simulink model "Dynamics"  (R2023a)
settings: Solver=FixedStepAuto  StartTime=0.0  StopTime=inf  FixedStep=0.001  EnableMultiTasking=on
libraries: sharedutil x32, sharedtransform x18, dspmtrx3 x12, matrix_library x6, simulink_extras x1, simulink x1
(part 1 of 6)
settings Model: VariantFading=off  Creator=Amir  LastModifiedBy=NGAI-LAPTOP
settings SolverCC: ZeroCrossAlgorithm=Adaptive  AutoInsertRateTranBlk=on
settings DataIOCC: LimitDataPoints=on  SaveFormat=Array  ReturnWorkspaceOutputs=off
settings OptimizationCC: LifeSpan=inf
settings DebuggingCC: UnconnectedInputMsg=warning  UnconnectedOutputMsg=warning  UnconnectedLineMsg=warning  SFUnexpectedBacktrackingDiag=warning  SFNoUnconditionalDefaultTransitionDiag=warning  SFExecutionAtInitializationDiag=none  ArithmeticOperatorsInVariantConditions=warning
settings HardwareCC: ProdBitPerPointer=32  ProdBitPerSizeT=32  ProdBitPerPtrDiffT=32  ProdLargestAtomicFloat=None  ProdIntDivRoundTo=Undefined  ProdEndianess=Unspecified  ProdWordSize=32  ProdHWDeviceType=32-bit Generic
settings ModelReferenceCC: PropagateSignalLabelsOutOfModel=off
settings SFSimCC: SimUseLocalCustomCode=off  CustomCodeUndefinedFunction=UseInterfaceOnly
settings RTWCC: RTWUseLocalCustomCode=off
settings CodeAppCC: StateflowObjectComments=on
settings GRTTargetCC: TargetLangStandard=C89/C90 (ANSI)
settings ConfigComp: CovMetricSettings=dw  CovSaveCumulativeToWorkspaceVar=on  CovSaveSingleToWorkspaceVar=on  CovExternalEMLEnable=off

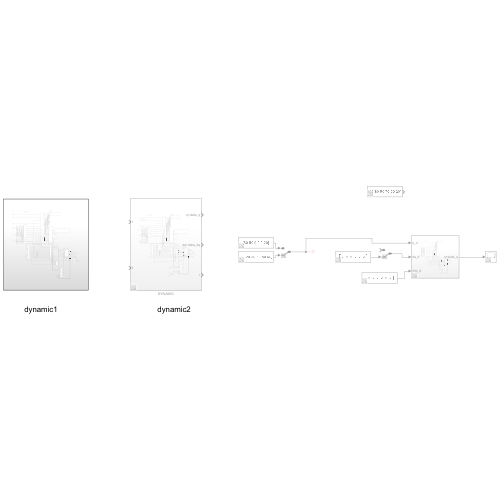
[thumbnail: Simulink's stored preview of the top-level diagram]
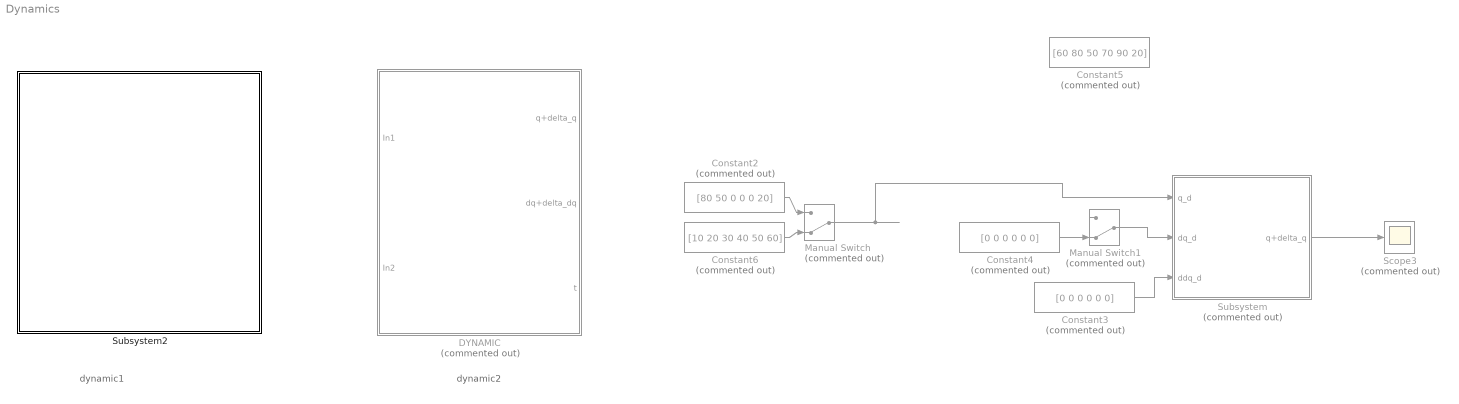
== system Dynamics ==
  note: dynamic1
  note: dynamic2
  Constant2 : Constant  Commented=on  Value=[80 50 0 0 0 20]
  Constant3 : Constant  Commented=on  Value=[0 0 0 0 0 0]
  Constant4 : Constant  Commented=on  Value=[0 0 0 0 0 0]
  Constant5 : Constant  Commented=on  Value=[60 80 50 70 90 20]
  Constant6 : Constant  Commented=on  Value=[10 20 30 40 50 60]
  DYNAMIC : Subsystem  Commented=on
  Manual Switch : ManualSwitch  Commented=on  CurrentSetting=0
  Manual Switch1 : ManualSwitch  Commented=on  CurrentSetting=0
  Scope3 : Scope  Commented=on
  Subsystem : Subsystem  Commented=on
  Subsystem2 : Subsystem
  wires:
  Subsystem/1(q+delta_q) -> Scope3/1
  Constant3/1 -> Subsystem/3(ddq_d)
  Constant2/1 -> Manual Switch/1
  Constant6/1 -> Manual Switch/2
  Manual Switch/1 -> Subsystem/1(q_d)
  Manual Switch1/1 -> Subsystem/2(dq_d)
  Constant4/1 -> Manual Switch1/2

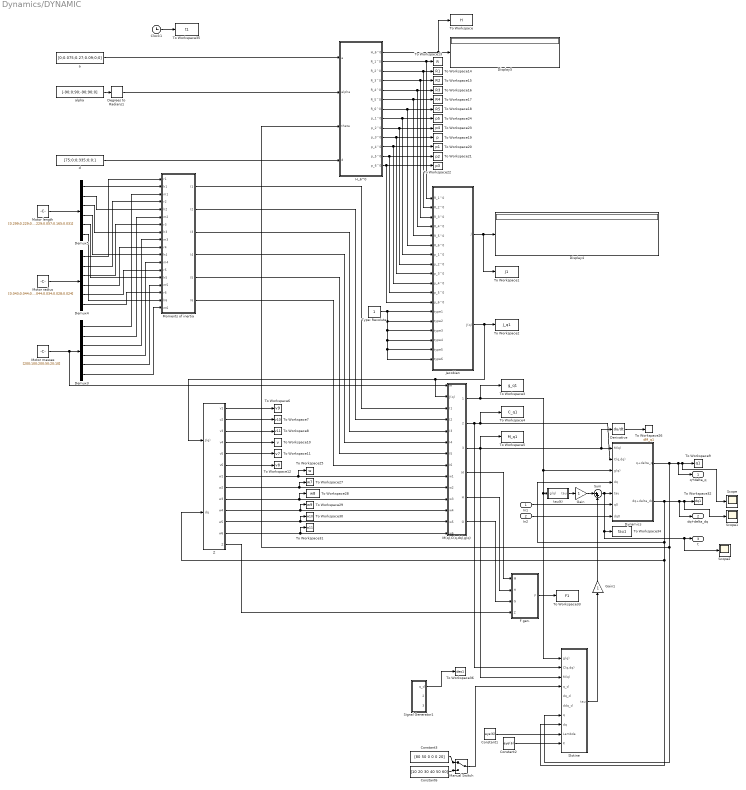
== system Dynamics/DYNAMIC ==
  In1 : Inport
  In2 : Inport  Port=2
  Clock1 : Clock
  Constant1 : Constant  Value=eye(6)
  Constant2 : Constant  Value=eye(6)
  Constant3 : Constant  Value=[80 50 0 0 0 20]
  Constant6 : Constant  Value=[10 20 30 40 50 60]
  Degrees to Radians1 : simulink_extras/Transformations/Degrees to Radians
  Demux3 : Demux  Outputs=6
  Demux4 : Demux  Outputs=6
  Demux5 : Demux  Outputs=6
  Derivative : Derivative
  Display4 : Display
  Display5 : Display
  Dynamics : Subsystem
  F gen. : Subsystem
  Gain : Gain
  Gain1 : Gain
  H_6^0 : Subsystem
  Jacobian : Subsystem
  M(q),C(q,dq),g(q) : Subsystem
  Manual Switch : ManualSwitch
  Moments of inertia : Subsystem
  Motor length : Constant  Value=[0.299;0.229;0.229;0.057;0.165;0.031]
  Motor masses : Constant  Value=[200;100;200;50;20;10]
  Motor radius : Constant  Value=[0.043;0.044;0.044;0.034;0.028;0.024]
  Scope : Scope
  Scope1 : Scope
  Scope2 : Scope
  Signal Generator1 : Subsystem
  Slotine : Subsystem
  Sum : Sum  Inputs=|++
  To Workspace : ToWorkspace  VariableName=H  SampleTime=-1
  To Workspace1 : ToWorkspace  VariableName=J1  SampleTime=-1
  To Workspace10 : ToWorkspace  VariableName=v  SampleTime=-1
  To Workspace11 : ToWorkspace  VariableName=v7  SampleTime=-1
  To Workspace12 : ToWorkspace  VariableName=v8  SampleTime=-1
  To Workspace13 : ToWorkspace  VariableName=R  SampleTime=-1
  To Workspace14 : ToWorkspace  VariableName=R1  SampleTime=-1
  To Workspace15 : ToWorkspace  VariableName=R2  SampleTime=-1
  To Workspace16 : ToWorkspace  VariableName=R3  SampleTime=-1
  To Workspace17 : ToWorkspace  VariableName=R4  SampleTime=-1
  To Workspace18 : ToWorkspace  VariableName=R5  SampleTime=-1
  To Workspace19 : ToWorkspace  VariableName=p  SampleTime=-1
  To Workspace2 : ToWorkspace  VariableName=J_q1  SampleTime=-1
  To Workspace20 : ToWorkspace  VariableName=p1  SampleTime=-1
  To Workspace21 : ToWorkspace  VariableName=p2  SampleTime=-1
  To Workspace22 : ToWorkspace  VariableName=p3  SampleTime=-1
  To Workspace23 : ToWorkspace  VariableName=p4  SampleTime=-1
  To Workspace24 : ToWorkspace  VariableName=p5  SampleTime=-1
  To Workspace25 : ToWorkspace  VariableName=w  SampleTime=-1
  To Workspace26 : ToWorkspace  VariableName=dM_q1  SampleTime=-1
  To Workspace27 : ToWorkspace  VariableName=w7  SampleTime=-1
  To Workspace28 : ToWorkspace  VariableName=w8  SampleTime=-1
  To Workspace29 : ToWorkspace  VariableName=w9  SampleTime=-1
  To Workspace3 : ToWorkspace  VariableName=g_q1  SampleTime=-1
  To Workspace30 : ToWorkspace  VariableName=w10  SampleTime=-1
  To Workspace31 : ToWorkspace  VariableName=w11  SampleTime=-1
  To Workspace32 : ToWorkspace  VariableName=dq1  SampleTime=-1
  To Workspace33 : ToWorkspace  VariableName=F1  SampleTime=-1
  To Workspace34 : ToWorkspace  VariableName=tau1  SampleTime=-1
  To Workspace35 : ToWorkspace  VariableName=t1  SampleTime=-1
  To Workspace36 : ToWorkspace  VariableName=des1  SampleTime=-1
  To Workspace4 : ToWorkspace  VariableName=C_q1  SampleTime=-1
  To Workspace5 : ToWorkspace  VariableName=M_q1  SampleTime=-1
  To Workspace6 : ToWorkspace  VariableName=v9  SampleTime=-1
  To Workspace7 : ToWorkspace  VariableName=v10  SampleTime=-1
  To Workspace8 : ToWorkspace  VariableName=v11  SampleTime=-1
  To Workspace9 : ToWorkspace  VariableName=q1  SampleTime=-1
  Type: Revolute : Constant
  Z : Subsystem
  a : Constant  Value=[0;0.075;0.27;0.09;0;0]
  alpha : Constant  Value=[-90;0;90;-90;90;0]
  d : Constant  Value=[75;0;0;335;0;0;]
  tau(t) : Subsystem
  q+delta_q : Outport
  dq+delta_dq : Outport  Port=2
  t : Outport  Port=3
  wires:
  Demux5/1 -> Moments of inertia/2(h1)
  Z/12(w6) -> To Workspace31/1, M(q),C(q,dq),g(q)/14(w6)
  Moments of inertia/6(I6) -> M(q),C(q,dq),g(q)/8(I6)
  Dynamics/2(dq+delta_dq) -> dq+delta_dq/1, Scope1/1, To Workspace32/1, Z/2(dq), Slotine/8(dq), Dynamics/4(dq)
  Z/11(w5) -> To Workspace30/1, M(q),C(q,dq),g(q)/13(w5)
  Moments of inertia/5(I5) -> M(q),C(q,dq),g(q)/7(I5)
  M(q),C(q,dq),g(q)/1(g(q)) -> Dynamics/3(g(q)), tau(t)/1(g(q)), Slotine/1(g(q)), To Workspace3/1
  Demux3/2 -> Moments of inertia/6(m2)
  Dynamics/1(q+delta_q) -> q+delta_q/1, Scope/1, To Workspace9/1, Slotine/7(q), H_6^0/3(theta)
  Moments of inertia/1(I1) -> M(q),C(q,dq),g(q)/3(I1)
  H_6^0/2(R_1^0) -> To Workspace13/1, Jacobian/1(R_1^0)
  In1/1 -> Dynamics/6(q0)
  Z/7(w1) -> To Workspace25/1, M(q),C(q,dq),g(q)/9(w1)
  Z/9(w3) -> To Workspace28/1, M(q),C(q,dq),g(q)/11(w3)
  Demux5/4 -> Moments of inertia/11(h4)
  Moments of inertia/4(I4) -> M(q),C(q,dq),g(q)/6(I4)
  Z/4(v4) -> To Workspace10/1
  H_6^0/12(p_5^0) -> To Workspace21/1, Jacobian/11(p_5^0)
  M(q),C(q,dq),g(q)/2(C(q,dq)) -> Slotine/2(C(q,dq)), To Workspace4/1, Dynamics/2(C(q,dq))
  Demux3/6 -> Moments of inertia/18(m6)
  Jacobian/2(J(q)) -> M(q),C(q,dq),g(q)/2(J(q)), Z/1(J(q)), To Workspace2/1
  H_6^0/11(p_4^0) -> To Workspace20/1, Jacobian/10(p_4^0)
  Demux3/3 -> Moments of inertia/9(m3)
  H_6^0/4(R_3^0) -> To Workspace15/1, Jacobian/3(R_3^0)
  Clock1/1 -> To Workspace35/1
  d/1 -> H_6^0/4(d)
  H_6^0/5(R_4^0) -> To Workspace16/1, Jacobian/4(R_4^0)
  Slotine/1(tau) -> Gain1/1
  Demux4/6 -> Moments of inertia/16(r6)
  H_6^0/1(H_6^0) -> To Workspace/1, Display5/1
  In2/1 -> Dynamics/7(dq0)
  H_6^0/8(p_1^0) -> Jacobian/7(p_1^0), To Workspace24/1
  Derivative/1 -> To Workspace26/1
  M(q),C(q,dq),g(q)/5(H) -> F gen./2(H)
  a/1 -> H_6^0/1(a)
  H_6^0/6(R_5^0) -> To Workspace17/1, Jacobian/5(R_5^0)
  Motor radius/1 -> Demux4/1
  Constant1/1 -> Slotine/9(Lambda)
  H_6^0/7(R_6^0) -> To Workspace18/1, Jacobian/6(R_6^0)
  H_6^0/9(p_2^0) -> To Workspace23/1, Jacobian/8(p_2^0)
  Signal Generator1/1(q_d) -> To Workspace36/1
  Demux3/1 -> Moments of inertia/3(m1)
  Demux5/3 -> Moments of inertia/8(h3)
  tau(t)/1(tau) -> Gain/1
  M(q),C(q,dq),g(q)/6(G) -> F gen./3(G)
  Degrees to Radians1/1 -> H_6^0/2(alpha)
  Sum/1 -> Scope2/1, t/1, To Workspace34/1, Dynamics/5(tau)
  Z/13(Z) -> F gen./4(Z)
  H_6^0/3(R_2^0) -> To Workspace14/1, Jacobian/2(R_2^0)
  Demux4/1 -> Moments of inertia/1(r1)
  Z/10(w4) -> To Workspace29/1, M(q),C(q,dq),g(q)/12(w4)
  Z/6(v6) -> To Workspace12/1
  H_6^0/13(p_6^0) -> To Workspace22/1, Jacobian/12(p_6^0)
  Moments of inertia/2(I2) -> M(q),C(q,dq),g(q)/4(I2)
  Motor length/1 -> Demux5/1
  Demux4/2 -> Moments of inertia/4(r2)
  Jacobian/1(J) -> To Workspace1/1, Display4/1
  Z/2(v2) -> To Workspace7/1
  H_6^0/10(p_3^0) -> Jacobian/9(p_3^0), To Workspace19/1
  Gain/1 -> Sum/1
  Demux3/5 -> Moments of inertia/15(m5)
  Demux5/6 -> Moments of inertia/17(h6)
  M(q),C(q,dq),g(q)/3(M(q)) -> Slotine/3(M(q)), To Workspace5/1, Derivative/1, Dynamics/1(M(q))
  M(q),C(q,dq),g(q)/4(M) -> F gen./1(M)
  Z/3(v3) -> To Workspace8/1
  Demux5/5 -> Moments of inertia/14(h5)
  F gen./1(F) -> To Workspace33/1
  Type: Revolute/1 -> Jacobian/14(type2), Jacobian/15(type3), Jacobian/18(type6), Jacobian/17(type5), Jacobian/16(type4), Jacobian/13(type1)
  Motor masses/1 -> Demux3/1, M(q),C(q,dq),g(q)/1(m)
  Z/8(w2) -> To Workspace27/1, M(q),C(q,dq),g(q)/10(w2)
  Z/1(v1) -> To Workspace6/1
  Gain1/1 -> Sum/2
  Moments of inertia/3(I3) -> M(q),C(q,dq),g(q)/5(I3)
  Demux4/3 -> Moments of inertia/7(r3)
  Demux4/5 -> Moments of inertia/13(r5)
  Z/5(v5) -> To Workspace11/1
  Demux4/4 -> Moments of inertia/10(r4)
  Demux3/4 -> Moments of inertia/12(m4)
  Constant2/1 -> Slotine/10(K)
  Demux5/2 -> Moments of inertia/5(h2)
  alpha/1 -> Degrees to Radians1/1
  Constant6/1 -> Manual Switch/2
  Constant3/1 -> Manual Switch/1
  Manual Switch/1 -> Slotine/4(q_d)

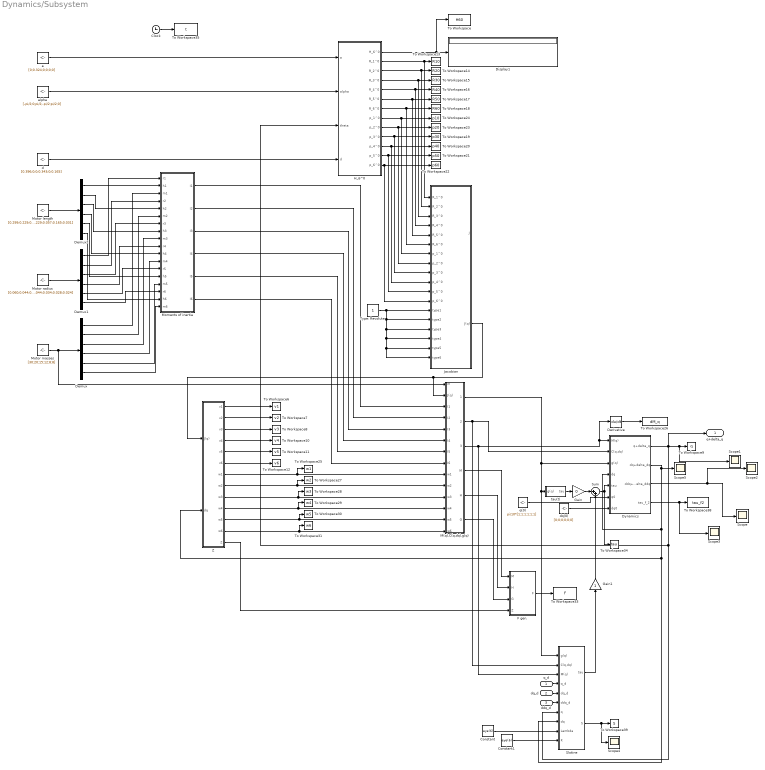
== system Dynamics/Subsystem ==
  q_d : Inport
  dq_d : Inport  Port=2
  ddq_d : Inport  Port=3
  Clock : Clock
  Constant : Constant  Value=eye(6)
  Constant1 : Constant  Value=eye(6)
  Demux : Demux  Outputs=6
  Demux1 : Demux  Outputs=6
  Demux2 : Demux  Outputs=6
  Derivative : Derivative
  Display1 : Display
  Dynamics : Subsystem
  F gen. : Subsystem
  Gain : Gain  Gain=0
  Gain1 : Gain
  H_6^0 : Subsystem
  Jacobian : Subsystem
  M(q),C(q,dq),g(q) : Subsystem
  Moments of inertia : Subsystem
  Motor length : Constant  Value=[0.299;0.229;0.229;0.057;0.165;0.031]
  Motor masses : Constant  Value=[30;20;15;12;8;8]
  Motor radius : Constant  Value=[0.060;0.044;0.044;0.034;0.028;0.024]
  Scope{,1..5} (6 alike) : Scope
  Slotine : Subsystem
  Sum : Sum  Inputs=|++
  To Workspace : ToWorkspace  VariableName=H60  SampleTime=-1
  To Workspace10 : ToWorkspace  VariableName=v4  SampleTime=-1
  To Workspace11 : ToWorkspace  VariableName=v5  SampleTime=-1
  To Workspace12 : ToWorkspace  VariableName=v6  SampleTime=-1
  To Workspace13 : ToWorkspace  VariableName=R10  SampleTime=-1
  To Workspace14 : ToWorkspace  VariableName=R20  SampleTime=-1
  To Workspace15 : ToWorkspace  VariableName=R30  SampleTime=-1
  To Workspace16 : ToWorkspace  VariableName=R40  SampleTime=-1
  To Workspace17 : ToWorkspace  VariableName=R50  SampleTime=-1
  To Workspace18 : ToWorkspace  VariableName=R60  SampleTime=-1
  To Workspace19 : ToWorkspace  VariableName=p30  SampleTime=-1
  To Workspace20 : ToWorkspace  VariableName=p40  SampleTime=-1
  To Workspace21 : ToWorkspace  VariableName=p50  SampleTime=-1
  To Workspace22 : ToWorkspace  VariableName=p60  SampleTime=-1
  To Workspace23 : ToWorkspace  VariableName=p20  SampleTime=-1
  To Workspace24 : ToWorkspace  VariableName=p10  SampleTime=-1
  To Workspace25 : ToWorkspace  VariableName=w1  SampleTime=-1
  To Workspace26 : ToWorkspace  VariableName=dM_q  SampleTime=-1
  To Workspace27 : ToWorkspace  VariableName=w2  SampleTime=-1
  To Workspace28 : ToWorkspace  VariableName=w3  SampleTime=-1
  To Workspace29 : ToWorkspace  VariableName=w4  SampleTime=-1
  To Workspace30 : ToWorkspace  VariableName=w5  SampleTime=-1
  To Workspace31 : ToWorkspace  VariableName=w6  SampleTime=-1
  To Workspace33 : ToWorkspace  VariableName=F  SampleTime=-1
  To Workspace34 : ToWorkspace  VariableName=tau  SampleTime=-1
  To Workspace35 : ToWorkspace  VariableName=t  SampleTime=-1
  To Workspace38 : ToWorkspace  VariableName=tau_f2  SampleTime=-1
  To Workspace39 : ToWorkspace  VariableName=S  SampleTime=-1
  To Workspace6 : ToWorkspace  VariableName=v1  SampleTime=-1
  To Workspace7 : ToWorkspace  VariableName=v2  SampleTime=-1
  To Workspace8 : ToWorkspace  VariableName=v3  SampleTime=-1
  To Workspace9 : ToWorkspace  VariableName=q  SampleTime=-1
  Type: Revolute : Constant
  Z : Subsystem
  a : Constant  Value=[0;0.324;0;0;0;0]
  alpha : Constant  Value=[-pi/2;0;pi/2;-pi/2;pi/2;0]
  d : Constant  Value=[0.396;0;0;0.343;0;0.165]
  dq(0) : Constant  Value=[0;0;0;0;0;0]
  q(0) : Constant  Value=pi/10*[1;1;1;1;1;1]
  tau(t) : Subsystem
  q+delta_q : Outport
  wires:
  Demux1/5 -> Moments of inertia/13(r5)
  H_6^0/10(p_3^0) -> Jacobian/9(p_3^0), To Workspace19/1
  Z/10(w4) -> To Workspace29/1, M(q),C(q,dq),g(q)/12(w4)
  Dynamics/4(tau_f_2) -> Scope3/1, To Workspace38/1
  M(q),C(q,dq),g(q)/1(g(q)) -> tau(t)/1(g(q)), Slotine/1(g(q)), Dynamics/3(g(q))
  M(q),C(q,dq),g(q)/3(M(q)) -> Slotine/3(M(q)), Derivative/1, Dynamics/1(M(q))
  Motor masses/1 -> M(q),C(q,dq),g(q)/1(m), Demux/1
  F gen./1(F) -> To Workspace33/1
  H_6^0/12(p_5^0) -> To Workspace21/1, Jacobian/11(p_5^0)
  Demux2/4 -> Moments of inertia/11(h4)
  alpha/1 -> H_6^0/2(alpha)
  Gain/1 -> Sum/1
  Dynamics/1(q+delta_q) -> H_6^0/3(theta), Slotine/7(q), q+delta_q/1, Scope1/1, To Workspace9/1
  Z/9(w3) -> To Workspace28/1, M(q),C(q,dq),g(q)/11(w3)
  Demux/1 -> Moments of inertia/3(m1)
  Slotine/2(S) -> Scope4/1, To Workspace39/1
  d/1 -> H_6^0/4(d)
  Demux2/5 -> Moments of inertia/14(h5)
  Dynamics/2(dq+delta_dq) -> Scope5/1, Slotine/8(dq), Z/2(dq), Dynamics/4(dq)
  Jacobian/2(J(q)) -> M(q),C(q,dq),g(q)/2(J(q)), Z/1(J(q))
  Constant1/1 -> Slotine/10(K)
  Z/3(v3) -> To Workspace8/1
  M(q),C(q,dq),g(q)/5(H) -> F gen./2(H)
  H_6^0/11(p_4^0) -> To Workspace20/1, Jacobian/10(p_4^0)
  Demux2/3 -> Moments of inertia/8(h3)
  H_6^0/8(p_1^0) -> Jacobian/7(p_1^0), To Workspace24/1
  Z/11(w5) -> To Workspace30/1, M(q),C(q,dq),g(q)/13(w5)
  tau(t)/1(tau) -> Gain/1
  Demux2/2 -> Moments of inertia/5(h2)
  H_6^0/1(H_6^0) -> To Workspace/1, Display1/1
  H_6^0/2(R_1^0) -> To Workspace13/1, Jacobian/1(R_1^0)
  H_6^0/13(p_6^0) -> To Workspace22/1, Jacobian/12(p_6^0)
  Z/7(w1) -> To Workspace25/1, M(q),C(q,dq),g(q)/9(w1)
  Sum/1 -> To Workspace34/1, Dynamics/5(tau)
  Moments of inertia/4(I4) -> M(q),C(q,dq),g(q)/6(I4)
  a/1 -> H_6^0/1(a)
  M(q),C(q,dq),g(q)/2(C(q,dq)) -> Slotine/2(C(q,dq)), Dynamics/2(C(q,dq))
  Demux1/3 -> Moments of inertia/7(r3)
  H_6^0/6(R_5^0) -> To Workspace17/1, Jacobian/5(R_5^0)
  dq_d/1 -> Slotine/5(dq_d)
  Moments of inertia/5(I5) -> M(q),C(q,dq),g(q)/7(I5)
  Demux2/1 -> Moments of inertia/2(h1)
  Z/8(w2) -> To Workspace27/1, M(q),C(q,dq),g(q)/10(w2)
  Moments of inertia/1(I1) -> M(q),C(q,dq),g(q)/3(I1)
  Demux1/4 -> Moments of inertia/10(r4)
  H_6^0/3(R_2^0) -> To Workspace14/1, Jacobian/2(R_2^0)
  Slotine/1(tau) -> Gain1/1
  Constant/1 -> Slotine/9(Lambda)
  Moments of inertia/3(I3) -> M(q),C(q,dq),g(q)/5(I3)
  H_6^0/9(p_2^0) -> To Workspace23/1, Jacobian/8(p_2^0)
  Demux1/2 -> Moments of inertia/4(r2)
  Demux2/6 -> Moments of inertia/17(h6)
  Z/12(w6) -> To Workspace31/1, M(q),C(q,dq),g(q)/14(w6)
  q(0)/1 -> Dynamics/6(q0)
  Moments of inertia/6(I6) -> M(q),C(q,dq),g(q)/8(I6)
  Demux1/6 -> Moments of inertia/16(r6)
  M(q),C(q,dq),g(q)/4(M) -> F gen./1(M)
  Z/6(v6) -> To Workspace12/1
  Demux/5 -> Moments of inertia/15(m5)
  Z/2(v2) -> To Workspace7/1
  Demux/3 -> Moments of inertia/9(m3)
  M(q),C(q,dq),g(q)/6(G) -> F gen./3(G)
  Demux/2 -> Moments of inertia/6(m2)
  Z/13(Z) -> F gen./4(Z)
  Motor length/1 -> Demux2/1
  Demux/6 -> Moments of inertia/18(m6)
  Moments of inertia/2(I2) -> M(q),C(q,dq),g(q)/4(I2)
  H_6^0/4(R_3^0) -> To Workspace15/1, Jacobian/3(R_3^0)
  Demux/4 -> Moments of inertia/12(m4)
  Z/4(v4) -> To Workspace10/1
  Derivative/1 -> To Workspace26/1
  H_6^0/5(R_4^0) -> To Workspace16/1, Jacobian/4(R_4^0)
  Z/1(v1) -> To Workspace6/1
  Clock/1 -> To Workspace35/1
  H_6^0/7(R_6^0) -> To Workspace18/1, Jacobian/6(R_6^0)
  ddq_d/1 -> Slotine/6(ddq_d)
  Type: Revolute/1 -> Jacobian/14(type2), Jacobian/15(type3), Jacobian/18(type6), Jacobian/17(type5), Jacobian/16(type4), Jacobian/13(type1)
  Z/5(v5) -> To Workspace11/1
  Gain1/1 -> Sum/2
  dq(0)/1 -> Dynamics/7(dq0)
  Demux1/1 -> Moments of inertia/1(r1)
  Motor radius/1 -> Demux1/1
  q_d/1 -> Slotine/4(q_d)
  Dynamics/3(ddq+delta_ddq) -> Scope/1, Scope2/1

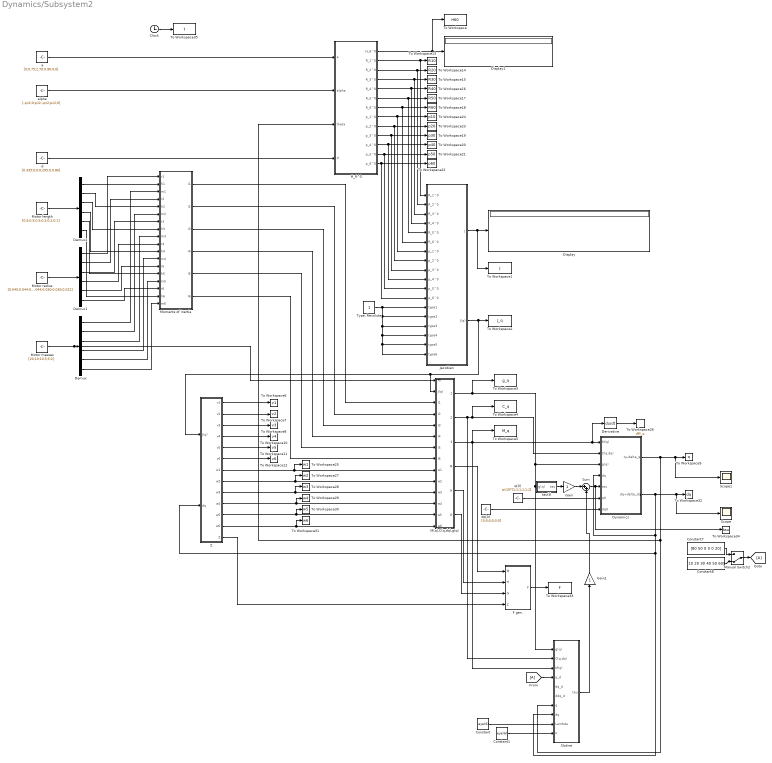
== system Dynamics/Subsystem2 ==
  Clock : Clock
  Constant : Constant  Value=eye(6)
  Constant1 : Constant  Value=eye(6)
  Constant7 : Constant  Value=[80 50 0 0 0 20]
  Constant8 : Constant  Value=[10 20 30 40 50 60]
  Demux : Demux  Outputs=6
  Demux1 : Demux  Outputs=6
  Demux2 : Demux  Outputs=6
  Derivative : Derivative
  Display : Display
  Display1 : Display
  Dynamics : Subsystem
  F gen. : Subsystem
  From : From
  Gain : Gain
  Gain1 : Gain
  Goto : Goto
  H_6^0 : Subsystem
  Jacobian : Subsystem
  M(q),C(q,dq),g(q) : Subsystem
  Manual Switch2 : ManualSwitch  CurrentSetting=0
  Moments of inertia : Subsystem
  Motor length : Constant  Value=[0.5;0.5;0.5;0.2;0.2;0.1]
  Motor masses : Constant  Value=[20;10;10;5;5;2]
  Motor radius : Constant  Value=[0.045;0.044;0.044;0.030;0.030;0.022]  VectorParams1D=off
  Scope : Scope
  Scope1 : Scope
  Slotine : Subsystem
  Sum : Sum  Inputs=|++
  To Workspace : ToWorkspace  VariableName=H60  SampleTime=-1
  To Workspace1 : ToWorkspace  VariableName=J  SampleTime=-1
  To Workspace10 : ToWorkspace  VariableName=v4  SampleTime=-1
  To Workspace11 : ToWorkspace  VariableName=v5  SampleTime=-1
  To Workspace12 : ToWorkspace  VariableName=v6  SampleTime=-1
  To Workspace13 : ToWorkspace  VariableName=R10  SampleTime=-1
  To Workspace14 : ToWorkspace  VariableName=R20  SampleTime=-1
  To Workspace15 : ToWorkspace  VariableName=R30  SampleTime=-1
  To Workspace16 : ToWorkspace  VariableName=R40  SampleTime=-1
  To Workspace17 : ToWorkspace  VariableName=R50  SampleTime=-1
  To Workspace18 : ToWorkspace  VariableName=R60  SampleTime=-1
  To Workspace19 : ToWorkspace  VariableName=p30  SampleTime=-1
  To Workspace2 : ToWorkspace  VariableName=J_q  SampleTime=-1
  To Workspace20 : ToWorkspace  VariableName=p40  SampleTime=-1
  To Workspace21 : ToWorkspace  VariableName=p50  SampleTime=-1
  To Workspace22 : ToWorkspace  VariableName=p60  SampleTime=-1
  To Workspace23 : ToWorkspace  VariableName=p20  SampleTime=-1
  To Workspace24 : ToWorkspace  VariableName=p10  SampleTime=-1
  To Workspace25 : ToWorkspace  VariableName=w1  SampleTime=-1
  To Workspace26 : ToWorkspace  VariableName=dM_q  SampleTime=-1
  To Workspace27 : ToWorkspace  VariableName=w2  SampleTime=-1
  To Workspace28 : ToWorkspace  VariableName=w3  SampleTime=-1
  To Workspace29 : ToWorkspace  VariableName=w4  SampleTime=-1
  To Workspace3 : ToWorkspace  VariableName=g_q  SampleTime=-1
  To Workspace30 : ToWorkspace  VariableName=w5  SampleTime=-1
  To Workspace31 : ToWorkspace  VariableName=w6  SampleTime=-1
  To Workspace32 : ToWorkspace  VariableName=dq  SampleTime=-1
  To Workspace33 : ToWorkspace  VariableName=F  SampleTime=-1
  To Workspace34 : ToWorkspace  VariableName=tau  SampleTime=-1
  To Workspace35 : ToWorkspace  VariableName=t  SampleTime=-1
  To Workspace4 : ToWorkspace  VariableName=C_q  SampleTime=-1
  To Workspace5 : ToWorkspace  VariableName=M_q  SampleTime=-1
  To Workspace6 : ToWorkspace  VariableName=v1  SampleTime=-1
  To Workspace7 : ToWorkspace  VariableName=v2  SampleTime=-1
  To Workspace8 : ToWorkspace  VariableName=v3  SampleTime=-1
  To Workspace9 : ToWorkspace  VariableName=q  SampleTime=-1
  Type: Revolute : Constant
  Z : Subsystem
  a : Constant  Value=[0;0.75;2.70;0.90;0;0]
  alpha : Constant  Value=[-pi/2;0;pi/2;-pi/2;pi/2;0]
  d : Constant  Value=[0.335;0;0;0.295;0;0.80]
  dq(0) : Constant  Value=[0;0;0;0;0;0]
  q(0) : Constant  Value=pi/10*[1;1;1;1;1;1]
  tau(t) : Subsystem
  wires:
  Demux2/1 -> Moments of inertia/2(h1)
  alpha/1 -> H_6^0/2(alpha)
  Z/12(w6) -> To Workspace31/1, M(q),C(q,dq),g(q)/14(w6)
  H_6^0/8(p_1^0) -> Jacobian/7(p_1^0), To Workspace24/1
  Demux/6 -> Moments of inertia/18(m6)
  H_6^0/2(R_1^0) -> To Workspace13/1, Jacobian/1(R_1^0)
  H_6^0/4(R_3^0) -> To Workspace15/1, Jacobian/3(R_3^0)
  Moments of inertia/4(I4) -> M(q),C(q,dq),g(q)/6(I4)
  H_6^0/6(R_5^0) -> To Workspace17/1, Jacobian/5(R_5^0)
  Moments of inertia/1(I1) -> M(q),C(q,dq),g(q)/3(I1)
  Jacobian/2(J(q)) -> Z/1(J(q)), M(q),C(q,dq),g(q)/2(J(q)), To Workspace2/1
  H_6^0/12(p_5^0) -> To Workspace21/1, Jacobian/11(p_5^0)
  Z/11(w5) -> To Workspace30/1, M(q),C(q,dq),g(q)/13(w5)
  Demux/2 -> Moments of inertia/6(m2)
  Moments of inertia/5(I5) -> M(q),C(q,dq),g(q)/7(I5)
  Type: Revolute/1 -> Jacobian/14(type2), Jacobian/15(type3), Jacobian/18(type6), Jacobian/17(type5), Jacobian/16(type4), Jacobian/13(type1)
  H_6^0/5(R_4^0) -> To Workspace16/1, Jacobian/4(R_4^0)
  Z/4(v4) -> To Workspace10/1
  Z/8(w2) -> To Workspace27/1, M(q),C(q,dq),g(q)/10(w2)
  tau(t)/1(tau) -> Gain/1
  H_6^0/1(H_6^0) -> To Workspace/1, Display1/1
  H_6^0/7(R_6^0) -> To Workspace18/1, Jacobian/6(R_6^0)
  H_6^0/9(p_2^0) -> To Workspace23/1, Jacobian/8(p_2^0)
  M(q),C(q,dq),g(q)/3(M(q)) -> Slotine/3(M(q)), To Workspace5/1, Derivative/1, Dynamics/1(M(q))
  Constant1/1 -> Slotine/10(K)
  Z/9(w3) -> To Workspace28/1, M(q),C(q,dq),g(q)/11(w3)
  Z/5(v5) -> To Workspace11/1
  Demux1/6 -> Moments of inertia/16(r6)
  F gen./1(F) -> To Workspace33/1
  Z/2(v2) -> To Workspace7/1
  d/1 -> H_6^0/4(d)
  H_6^0/10(p_3^0) -> Jacobian/9(p_3^0), To Workspace19/1
  Demux1/2 -> Moments of inertia/4(r2)
  H_6^0/13(p_6^0) -> To Workspace22/1, Jacobian/12(p_6^0)
  M(q),C(q,dq),g(q)/6(G) -> F gen./3(G)
  Moments of inertia/2(I2) -> M(q),C(q,dq),g(q)/4(I2)
  H_6^0/11(p_4^0) -> To Workspace20/1, Jacobian/10(p_4^0)
  M(q),C(q,dq),g(q)/4(M) -> F gen./1(M)
  Z/7(w1) -> To Workspace25/1, M(q),C(q,dq),g(q)/9(w1)
  Demux/4 -> Moments of inertia/12(m4)
  Dynamics/2(dq+delta_dq) -> Scope/1, To Workspace32/1, Z/2(dq), Slotine/8(dq), Dynamics/4(dq)
  q(0)/1 -> Dynamics/6(q0)
  dq(0)/1 -> Dynamics/7(dq0)
  M(q),C(q,dq),g(q)/2(C(q,dq)) -> Slotine/2(C(q,dq)), To Workspace4/1, Dynamics/2(C(q,dq))
  Motor radius/1 -> Demux1/1
  Dynamics/1(q+delta_q) -> Scope1/1, To Workspace9/1, Slotine/7(q), H_6^0/3(theta)
  Z/6(v6) -> To Workspace12/1
  Demux/3 -> Moments of inertia/9(m3)
  Z/1(v1) -> To Workspace6/1
  Moments of inertia/6(I6) -> M(q),C(q,dq),g(q)/8(I6)
  Derivative/1 -> To Workspace26/1
  Jacobian/1(J) -> To Workspace1/1, Display/1
  Demux1/5 -> Moments of inertia/13(r5)
  Demux2/4 -> Moments of inertia/11(h4)
  a/1 -> H_6^0/1(a)
  Demux1/3 -> Moments of inertia/7(r3)
  Moments of inertia/3(I3) -> M(q),C(q,dq),g(q)/5(I3)
  Demux2/5 -> Moments of inertia/14(h5)
  Demux2/2 -> Moments of inertia/5(h2)
  Motor length/1 -> Demux2/1
  Z/10(w4) -> To Workspace29/1, M(q),C(q,dq),g(q)/12(w4)
  Clock/1 -> To Workspace35/1
  M(q),C(q,dq),g(q)/5(H) -> F gen./2(H)
  Demux/1 -> Moments of inertia/3(m1)
  M(q),C(q,dq),g(q)/1(g(q)) -> Dynamics/3(g(q)), tau(t)/1(g(q)), Slotine/1(g(q)), To Workspace3/1
  Demux1/1 -> Moments of inertia/1(r1)
  Demux1/4 -> Moments of inertia/10(r4)
  Z/3(v3) -> To Workspace8/1
  Demux2/6 -> Moments of inertia/17(h6)
  H_6^0/3(R_2^0) -> To Workspace14/1, Jacobian/2(R_2^0)
  Motor masses/1 -> Demux/1, M(q),C(q,dq),g(q)/1(m)
  Sum/1 -> To Workspace34/1, Dynamics/5(tau)
  Slotine/1(tau) -> Gain1/1
  Demux2/3 -> Moments of inertia/8(h3)
  Constant/1 -> Slotine/9(Lambda)
  Gain1/1 -> Sum/2
  Gain/1 -> Sum/1
  Demux/5 -> Moments of inertia/15(m5)
  Z/13(Z) -> F gen./4(Z)
  Constant8/1 -> Manual Switch2/2
  Constant7/1 -> Manual Switch2/1
  From/1 -> Slotine/4(q_d)
  Manual Switch2/1 -> Goto/1

== system Dynamics/DYNAMIC/Dynamics ==
  M(q) : Inport
  C(q,dq) : Inport  Port=2
  g(q) : Inport  Port=3
  dq : Inport  Port=4
  tau : Inport  Port=5
  q0 : Inport  Port=6
  dq0 : Inport  Port=7
  Add : Sum
  Add1 : Sum
  Gain : Gain  Gain=-1
  "Integrator, Second-Order" : SecondOrderIntegrator  ICSourceX=external  ICSourceDXDT=external
  Interpreted MATLAB Function : MATLABFcn  MATLABFcn=inv  OutputSignalType=real  Output1D=off
  Product : Product  Multiplication=Matrix(*)
  Product1 : Product  Multiplication=Matrix(*)
  q+delta_q : Outport
  dq+delta_dq : Outport  Port=2
  wires:
  C(q,dq)/1 -> Product/1
  dq/1 -> Product/2
  Product/1 -> Add/1
  g(q)/1 -> Add/2
  Add/1 -> Gain/1
  M(q)/1 -> Interpreted MATLAB Function/1
  Interpreted MATLAB Function/1 -> Product1/1
  Gain/1 -> Add1/1
  tau/1 -> Add1/2
  Add1/1 -> Product1/2
  Product1/1 -> "Integrator, Second-Order"/1
  "Integrator, Second-Order"/2 -> dq+delta_dq/1
  "Integrator, Second-Order"/1 -> q+delta_q/1
  q0/1 -> "Integrator, Second-Order"/2
  dq0/1 -> "Integrator, Second-Order"/3

== system Dynamics/DYNAMIC/F gen. ==
  M : Inport
  H : Inport  Port=2
  G : Inport  Port=3
  Z : Inport  Port=4
  Add : Sum  Inputs=+++
  Derivative : Derivative
  Product1 : Product  Multiplication=Matrix(*)
  Product2 : Product  Multiplication=Matrix(*)
  F : Outport
  wires:
  Z/1 -> Product1/2, Derivative/1
  Add/1 -> F/1
  G/1 -> Add/3
  Product2/1 -> Add/1
  M/1 -> Product2/1
  Derivative/1 -> Product2/2
  Product1/1 -> Add/2
  H/1 -> Product1/1

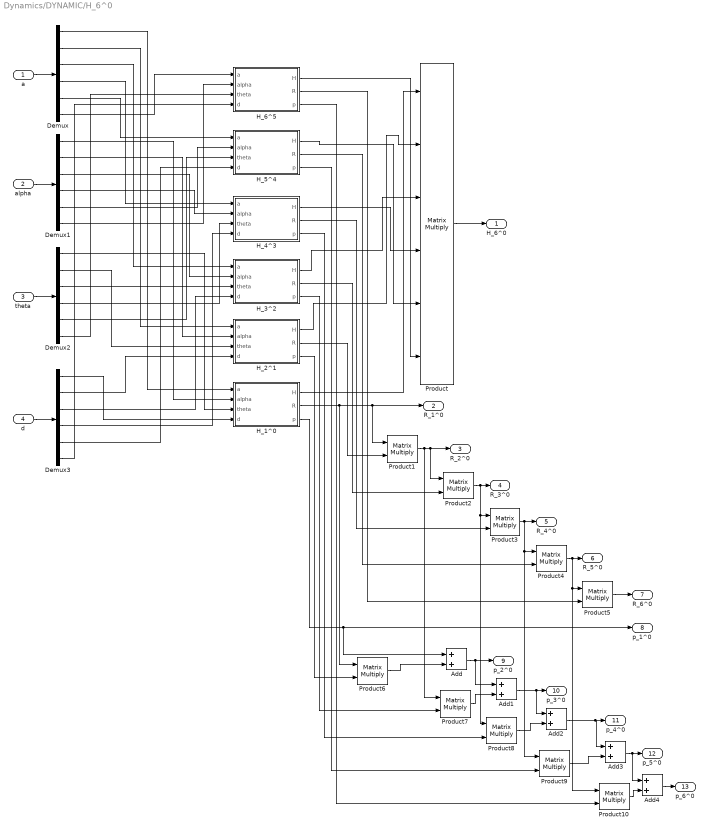
== system Dynamics/DYNAMIC/H_6^0 ==
  a : Inport
  alpha : Inport  Port=2
  theta : Inport  Port=3
  d : Inport  Port=4
  Add{,1..4} (5 alike) : Sum
  Demux{,1..3} (4 alike) : Demux  Outputs=6
  H_1^0 : Subsystem
  H_2^1 : Subsystem
  H_3^2 : Subsystem
  H_4^3 : Subsystem
  H_5^4 : Subsystem
  H_6^5 : Subsystem
  Product : Product  Inputs=6  Multiplication=Matrix(*)
  Product{1..10} (10 alike) : Product  Multiplication=Matrix(*)
  H_6^0 : Outport
  R_1^0 : Outport  Port=2
  R_2^0 : Outport  Port=3
  R_3^0 : Outport  Port=4
  R_4^0 : Outport  Port=5
  R_5^0 : Outport  Port=6
  R_6^0 : Outport  Port=7
  p_1^0 : Outport  Port=8
  p_2^0 : Outport  Port=9
  p_3^0 : Outport  Port=10
  p_4^0 : Outport  Port=11
  p_5^0 : Outport  Port=12
  p_6^0 : Outport  Port=13
  wires:
  H_6^5/1(H) -> Product/6
  H_5^4/1(H) -> Product/5
  H_2^1/1(H) -> Product/2
  H_1^0/1(H) -> Product/1
  Product/1 -> H_6^0/1
  a/1 -> Demux/1
  d/1 -> Demux3/1
  H_4^3/1(H) -> Product/4
  H_3^2/1(H) -> Product/3
  Product1/1 -> Product7/1, Product2/1, R_2^0/1
  H_2^1/2(R) -> Product1/2
  Product2/1 -> Product8/1, Product3/1, R_3^0/1
  Product3/1 -> Product9/1, Product4/1, R_4^0/1
  Product4/1 -> Product10/1, Product5/1, R_5^0/1
  Product5/1 -> R_6^0/1
  Add/1 -> Add1/1, p_2^0/1
  theta/1 -> Demux2/1
  alpha/1 -> Demux1/1
  Demux/1 -> H_1^0/1(a)
  Demux/6 -> H_6^5/1(a)
  Demux/5 -> H_5^4/1(a)
  Demux/4 -> H_4^3/1(a)
  Demux/3 -> H_3^2/1(a)
  Demux/2 -> H_2^1/1(a)
  Demux1/6 -> H_6^5/2(alpha)
  Demux1/5 -> H_5^4/2(alpha)
  Demux1/4 -> H_4^3/2(alpha)
  Demux1/3 -> H_3^2/2(alpha)
  Demux1/2 -> H_2^1/2(alpha)
  Demux1/1 -> H_1^0/2(alpha)
  Demux2/6 -> H_6^5/3(theta)
  Demux2/5 -> H_5^4/3(theta)
  Demux2/4 -> H_4^3/3(theta)
  Demux2/3 -> H_3^2/3(theta)
  Demux2/2 -> H_2^1/3(theta)
  Demux2/1 -> H_1^0/3(theta)
  Demux3/1 -> H_1^0/4(d)
  Demux3/2 -> H_2^1/4(d)
  Demux3/3 -> H_3^2/4(d)
  Demux3/4 -> H_4^3/4(d)
  Demux3/5 -> H_5^4/4(d)
  Demux3/6 -> H_6^5/4(d)
  H_3^2/2(R) -> Product2/2
  H_4^3/2(R) -> Product3/2
  H_5^4/2(R) -> Product4/2
  H_6^5/2(R) -> Product5/2
  H_1^0/3(p) -> Add/1, p_1^0/1
  H_2^1/3(p) -> Product6/2
  Add1/1 -> Add2/1, p_3^0/1
  H_3^2/3(p) -> Product7/2
  H_4^3/3(p) -> Product8/2
  Add2/1 -> Add3/1, p_4^0/1
  H_5^4/3(p) -> Product9/2
  Add3/1 -> Add4/1, p_5^0/1
  H_6^5/3(p) -> Product10/2
  Add4/1 -> p_6^0/1
  H_1^0/2(R) -> R_1^0/1, Product1/1, Product6/1
  Product6/1 -> Add/2
  Product7/1 -> Add1/2
  Product8/1 -> Add2/2
  Product9/1 -> Add3/2
  Product10/1 -> Add4/2

== system Dynamics/DYNAMIC/Jacobian ==
  R_1^0 : Inport
  R_2^0 : Inport  Port=2
  R_3^0 : Inport  Port=3
  R_4^0 : Inport  Port=4
  R_5^0 : Inport  Port=5
  R_6^0 : Inport  Port=6
  p_1^0 : Inport  Port=7
  p_2^0 : Inport  Port=8
  p_3^0 : Inport  Port=9
  p_4^0 : Inport  Port=10
  p_5^0 : Inport  Port=11
  p_6^0 : Inport  Port=12
  type1 : Inport  Port=13
  type2 : Inport  Port=14
  type3 : Inport  Port=15
  type4 : Inport  Port=16
  type5 : Inport  Port=17
  type6 : Inport  Port=18
  J(q) gen. : Subsystem
  J_v : Subsystem
  J_w : Subsystem
  Vector Concatenate : Concatenate  Mode=Multidimensional array
  J : Outport
  J(q) : Outport  Port=2
  wires:
  R_1^0/1 -> J_v/1(R_1^0), J_w/1(R_1^0), J(q) gen./1(R_1^0)
  p_1^0/1 -> J_v/7(p_1^0), J(q) gen./7(p_1^0)
  p_2^0/1 -> J_v/8(p_2^0), J(q) gen./8(p_2^0)
  p_3^0/1 -> J_v/9(p_3^0), J(q) gen./9(p_3^0)
  p_4^0/1 -> J_v/10(p_4^0), J(q) gen./10(p_4^0)
  p_5^0/1 -> J_v/11(p_5^0), J(q) gen./11(p_5^0)
  R_2^0/1 -> J_v/2(R_2^0), J_w/2(R_2^0), J(q) gen./2(R_2^0)
  R_3^0/1 -> J_v/3(R_3^0), J_w/3(R_3^0), J(q) gen./3(R_3^0)
  R_4^0/1 -> J_v/4(R_4^0), J_w/4(R_4^0), J(q) gen./4(R_4^0)
  R_5^0/1 -> J_v/5(R_5^0), J_w/5(R_5^0), J(q) gen./5(R_5^0)
  type1/1 -> J_w/7(type1), J_v/13(type1), J(q) gen./12(type1)
  type2/1 -> J_w/8(type2), J(q) gen./13(type2), J_v/14(type2)
  type3/1 -> J_w/9(type3), J(q) gen./14(type3), J_v/15(type3)
  type4/1 -> J_w/10(type4), J(q) gen./15(type4), J_v/16(type4)
  type5/1 -> J_w/11(type5), J_v/17(type5)
  type6/1 -> J_w/12(type6), J_v/18(type6)
  p_6^0/1 -> J_v/12(p_6^0)
  J_v/1(J_v) -> J(q) gen./16(J_v_6(q)), Vector Concatenate/1
  J_w/1(EF J_w) -> Vector Concatenate/2
  Vector Concatenate/1 -> J/1
  J(q) gen./1(J(q)) -> J(q)/1
  J_w/2(J_w1) -> J(q) gen./17(J_w1)
  J_w/3(J_w2) -> J(q) gen./18(J_w2)
  J_w/4(J_w3) -> J(q) gen./19(J_w3)
  J_w/5(J_w4) -> J(q) gen./20(J_w4)
  J_w/6(J_w5) -> J(q) gen./21(J_w5)
  J_w/7(J_w6) -> J(q) gen./22(J_w6)
  R_6^0/1 -> J_v/6(R_6^0), J_w/6(R_6^0), J(q) gen./6(R_6^0)

== system Dynamics/DYNAMIC/M(q),C(q,dq),g(q) ==
  m : Inport
  J(q) : Inport  Port=2
  I1 : Inport  Port=3
  I2 : Inport  Port=4
  I3 : Inport  Port=5
  I4 : Inport  Port=6
  I5 : Inport  Port=7
  I6 : Inport  Port=8
  w1 : Inport  Port=9
  w2 : Inport  Port=10
  w3 : Inport  Port=11
  w4 : Inport  Port=12
  w5 : Inport  Port=13
  w6 : Inport  Port=14
  Add : Sum
  G gen : Subsystem
  Interpreted MATLAB Function : MATLABFcn  MATLABFcn=transpose  OutputSignalType=real  Output1D=off
  M,H : Subsystem
  Product{,1..3} (4 alike) : Product  Multiplication=Matrix(*)
  Product4 : Product  Inputs=3  Multiplication=Matrix(*)
  dJ : Derivative
  g(q) : Outport
  C(q,dq) : Outport  Port=2
  M(q) : Outport  Port=3
  M : Outport  Port=4
  H : Outport  Port=5
  G : Outport  Port=6
  wires:
  J(q)/1 -> Interpreted MATLAB Function/1, Product4/3, Product2/2, dJ/1
  Interpreted MATLAB Function/1 -> Product4/1, Product3/1, Product/1
  Product/1 -> g(q)/1
  m/1 -> G gen/1(m), M,H/1(m)
  I1/1 -> M,H/2(I1)
  I2/1 -> M,H/3(I2)
  I3/1 -> M,H/4(I3)
  I4/1 -> M,H/5(I4)
  I5/1 -> M,H/6(I5)
  I6/1 -> M,H/7(I6)
  w1/1 -> M,H/8(w1)
  w2/1 -> M,H/9(w2)
  w3/1 -> M,H/10(w3)
  w4/1 -> M,H/11(w4)
  w5/1 -> M,H/12(w5)
  w6/1 -> M,H/13(w6)
  M,H/1(M) -> Product1/1, M/1, Product4/2
  dJ/1 -> Product1/2
  M,H/2(H) -> H/1, Product2/1
  Product1/1 -> Add/1
  Product2/1 -> Add/2
  Add/1 -> Product3/2
  Product3/1 -> C(q,dq)/1
  Product4/1 -> M(q)/1
  G gen/1(G) -> G/1, Product/2

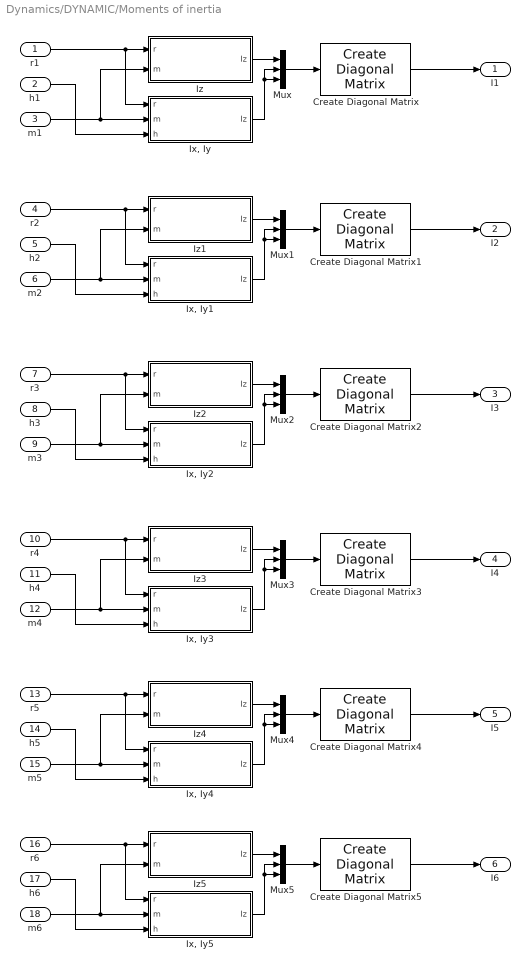
== system Dynamics/DYNAMIC/Moments of inertia ==
  r1 : Inport
  h1 : Inport  Port=2
  m1 : Inport  Port=3
  r2 : Inport  Port=4
  h2 : Inport  Port=5
  m2 : Inport  Port=6
  r3 : Inport  Port=7
  h3 : Inport  Port=8
  m3 : Inport  Port=9
  r4 : Inport  Port=10
  h4 : Inport  Port=11
  m4 : Inport  Port=12
  r5 : Inport  Port=13
  h5 : Inport  Port=14
  m5 : Inport  Port=15
  r6 : Inport  Port=16
  h6 : Inport  Port=17
  m6 : Inport  Port=18
  Create Diagonal Matrix{,1..5} (6 alike) : dspmtrx3/Create Diagonal Matrix
  "Ix, Iy" : Subsystem
  "Ix, Iy1" : Subsystem
  "Ix, Iy2" : Subsystem
  "Ix, Iy3" : Subsystem
  "Ix, Iy4" : Subsystem
  "Ix, Iy5" : Subsystem
  Iz : Subsystem
  Iz1 : Subsystem
  Iz2 : Subsystem
  Iz3 : Subsystem
  Iz4 : Subsystem
  Iz5 : Subsystem
  Mux{,1..5} (6 alike) : Mux  Inputs=3
  I1 : Outport
  I2 : Outport  Port=2
  I3 : Outport  Port=3
  I4 : Outport  Port=4
  I5 : Outport  Port=5
  I6 : Outport  Port=6
  wires:
  r1/1 -> "Ix, Iy"/1(r), Iz/1(r)
  m1/1 -> "Ix, Iy"/2(m), Iz/2(m)
  h1/1 -> "Ix, Iy"/3(h)
  Mux/1 -> Create Diagonal Matrix/1
  Iz/1(Iz) -> Mux/1
  "Ix, Iy"/1(Iz) -> Mux/3, Mux/2
  Create Diagonal Matrix/1 -> I1/1
  r2/1 -> "Ix, Iy1"/1(r), Iz1/1(r)
  m2/1 -> "Ix, Iy1"/2(m), Iz1/2(m)
  h2/1 -> "Ix, Iy1"/3(h)
  Mux1/1 -> Create Diagonal Matrix1/1
  Iz1/1(Iz) -> Mux1/1
  "Ix, Iy1"/1(Iz) -> Mux1/3, Mux1/2
  Create Diagonal Matrix1/1 -> I2/1
  r3/1 -> "Ix, Iy2"/1(r), Iz2/1(r)
  m3/1 -> "Ix, Iy2"/2(m), Iz2/2(m)
  h3/1 -> "Ix, Iy2"/3(h)
  Mux2/1 -> Create Diagonal Matrix2/1
  Iz2/1(Iz) -> Mux2/1
  "Ix, Iy2"/1(Iz) -> Mux2/3, Mux2/2
  Create Diagonal Matrix2/1 -> I3/1
  r4/1 -> "Ix, Iy3"/1(r), Iz3/1(r)
  m4/1 -> "Ix, Iy3"/2(m), Iz3/2(m)
  h4/1 -> "Ix, Iy3"/3(h)
  Mux3/1 -> Create Diagonal Matrix3/1
  Iz3/1(Iz) -> Mux3/1
  "Ix, Iy3"/1(Iz) -> Mux3/3, Mux3/2
  Create Diagonal Matrix3/1 -> I4/1
  r5/1 -> "Ix, Iy4"/1(r), Iz4/1(r)
  m5/1 -> "Ix, Iy4"/2(m), Iz4/2(m)
  h5/1 -> "Ix, Iy4"/3(h)
  Mux4/1 -> Create Diagonal Matrix4/1
  Iz4/1(Iz) -> Mux4/1
  "Ix, Iy4"/1(Iz) -> Mux4/3, Mux4/2
  Create Diagonal Matrix4/1 -> I5/1
  r6/1 -> "Ix, Iy5"/1(r), Iz5/1(r)
  m6/1 -> "Ix, Iy5"/2(m), Iz5/2(m)
  h6/1 -> "Ix, Iy5"/3(h)
  Mux5/1 -> Create Diagonal Matrix5/1
  Iz5/1(Iz) -> Mux5/1
  "Ix, Iy5"/1(Iz) -> Mux5/3, Mux5/2
  Create Diagonal Matrix5/1 -> I6/1

== system Dynamics/DYNAMIC/Signal Generator1 ==
  Add : Sum
  Clock{,1..5} (6 alike) : Clock
  Constant : Constant  Value=0.2
  Constant1 : Constant  Value=0.2
  Constant2 : Constant  Value=0.2
  Gain : Gain  Gain=-1
  Gain1 : Gain  Gain=-1
  Gain2 : Gain  Gain=-1
  Mux : Mux
  Mux1 : Mux
  Mux2 : Mux
  Product : Product
  Product1 : Product
  Product2 : Product
  Trigonometric Function : Trigonometry
  Trigonometric Function1 : Trigonometry  Operator=cos
  Trigonometric Function2 : Trigonometry  Operator=cos
  Trigonometric Function3 : Trigonometry
  Trigonometric Function4 : Trigonometry
  Trigonometric Function5 : Trigonometry  Operator=cos
  zeros(3,1) : Constant  Value=zeros(3,1)
  zeros(3,1)1 : Constant  Value=zeros(3,1)
  zeros(3,1)2 : Constant  Value=zeros(3,1)
  q_d : Outport
  dq_d : Outport  Port=2
  ddq_d : Outport  Port=3
  wires:
  Constant/1 -> Add/2, Product/1
  Trigonometric Function/1 -> Product/2
  Product/1 -> Mux/4, Mux/3
  Trigonometric Function1/1 -> Add/1
  Mux/1 -> q_d/1
  Add/1 -> Mux/2
  zeros(3,1)/1 -> Mux/1
  Clock/1 -> Trigonometric Function/1
  Clock1/1 -> Trigonometric Function1/1
  Constant1/1 -> Product1/1
  Trigonometric Function2/1 -> Product1/2
  Product1/1 -> Mux1/4, Mux1/3
  Mux1/1 -> dq_d/1
  Trigonometric Function3/1 -> Gain/1
  zeros(3,1)1/1 -> Mux1/1
  Clock2/1 -> Trigonometric Function2/1
  Clock3/1 -> Trigonometric Function3/1
  Gain/1 -> Mux1/2
  Constant2/1 -> Product2/1
  Product2/1 -> Gain2/1
  Mux2/1 -> ddq_d/1
  Trigonometric Function5/1 -> Gain1/1
  zeros(3,1)2/1 -> Mux2/1
  Clock4/1 -> Trigonometric Function4/1
  Clock5/1 -> Trigonometric Function5/1
  Gain1/1 -> Mux2/2
  Trigonometric Function4/1 -> Product2/2
  Gain2/1 -> Mux2/4, Mux2/3

== system Dynamics/DYNAMIC/Slotine ==
  g(q) : Inport
  C(q,dq) : Inport  Port=2
  M(q) : Inport  Port=3
  q_d : Inport  Port=4
  dq_d : Inport  Port=5
  ddq_d : Inport  Port=6
  q : Inport  Port=7
  dq : Inport  Port=8
  Lambda : Inport  Port=9
  K : Inport  Port=10
  S-gen : Subsystem
  V-gen : Subsystem
  dV-gen : Subsystem
  dq_tilde : Sum  Inputs=-+
  q_tilde : Sum  Inputs=-+
  tau-gen : Subsystem
  tau : Outport
  wires:
  q_d/1 -> q_tilde/1
  q/1 -> q_tilde/2
  dq_d/1 -> V-gen/2(dq_d), dq_tilde/1
  dq/1 -> S-gen/1(dq), dq_tilde/2
  ddq_d/1 -> dV-gen/2(ddq_d)
  q_tilde/1 -> V-gen/1(q_tilde)
  Lambda/1 -> dV-gen/3(Gamma), V-gen/3(Gamma)
  dq_tilde/1 -> dV-gen/1(dq_tilde)
  V-gen/1(V) -> tau-gen/4(V), S-gen/2(V)
  M(q)/1 -> tau-gen/1(M)
  C(q,dq)/1 -> tau-gen/2(C)
  g(q)/1 -> tau-gen/3(g)
  dV-gen/1(dV) -> tau-gen/5(dV)
  S-gen/1(S) -> tau-gen/6(S)
  K/1 -> tau-gen/7(K)
  tau-gen/1(tau) -> tau/1

== system Dynamics/DYNAMIC/Z ==
  J(q) : Inport
  dq : Inport  Port=2
  Demux : Demux  Outputs=36
  Mux{,1..11} (12 alike) : Mux  Inputs=3
  Product : Product  Multiplication=Matrix(*)
  v1 : Outport
  v2 : Outport  Port=2
  v3 : Outport  Port=3
  v4 : Outport  Port=4
  v5 : Outport  Port=5
  v6 : Outport  Port=6
  w1 : Outport  Port=7
  w2 : Outport  Port=8
  w3 : Outport  Port=9
  w4 : Outport  Port=10
  w5 : Outport  Port=11
  w6 : Outport  Port=12
  Z : Outport  Port=13
  wires:
  J(q)/1 -> Product/1
  dq/1 -> Product/2
  Product/1 -> Z/1, Demux/1
  Demux/1 -> Mux/1
  Demux/2 -> Mux/2
  Demux/3 -> Mux/3
  Mux/1 -> v1/1
  Demux/4 -> Mux1/1
  Demux/5 -> Mux1/2
  Demux/6 -> Mux1/3
  Mux1/1 -> v2/1
  Mux2/1 -> v3/1
  Demux/7 -> Mux2/1
  Demux/8 -> Mux2/2
  Demux/9 -> Mux2/3
  Mux3/1 -> v4/1
  Demux/10 -> Mux3/1
  Demux/11 -> Mux3/2
  Demux/12 -> Mux3/3
  Mux4/1 -> v5/1
  Demux/14 -> Mux4/2
  Demux/13 -> Mux4/1
  Demux/15 -> Mux4/3
  Mux5/1 -> v6/1
  Demux/17 -> Mux5/2
  Demux/16 -> Mux5/1
  Demux/18 -> Mux5/3
  Mux6/1 -> w1/1
  Demux/19 -> Mux6/1
  Demux/20 -> Mux6/2
  Demux/21 -> Mux6/3
  Mux7/1 -> w2/1
  Demux/22 -> Mux7/1
  Demux/23 -> Mux7/2
  Demux/24 -> Mux7/3
  Mux8/1 -> w3/1
  Demux/25 -> Mux8/1
  Demux/26 -> Mux8/2
  Demux/27 -> Mux8/3
  Mux9/1 -> w4/1
  Demux/28 -> Mux9/1
  Demux/29 -> Mux9/2
  Demux/30 -> Mux9/3
  Mux10/1 -> w5/1
  Demux/31 -> Mux10/1
  Demux/32 -> Mux10/2
  Demux/33 -> Mux10/3
  Mux11/1 -> w6/1
  Demux/34 -> Mux11/1
  Demux/35 -> Mux11/2
  Demux/36 -> Mux11/3

== system Dynamics/DYNAMIC/tau(t) ==
  g(q) : Inport
  Add : Sum
  Constant : Constant  Value=zeros(5,1)
  Gain : Gain  Gain=0
  Mux : Mux  Inputs=2
  Sine Wave : Sin  SampleTime=0
  tau : Outport
  wires:
  Sine Wave/1 -> Mux/2
  Constant/1 -> Mux/1
  Add/1 -> tau/1
  Mux/1 -> Gain/1
  g(q)/1 -> Add/1
  Gain/1 -> Add/2

== system Dynamics/Subsystem/Dynamics ==
  M(q) : Inport
  C(q,dq) : Inport  Port=2
  g(q) : Inport  Port=3
  dq : Inport  Port=4
  tau : Inport  Port=5
  q0 : Inport  Port=6
  dq0 : Inport  Port=7
  Add : Sum
  Add1 : Sum
  Band-Limited White Noise : simulink/Sources/Band-Limited White Noise  Cov=[0.1]  Ts=0.001  seed=[23341]
  Friction : Subsystem
  Gain : Gain  Gain=-1
  Gain1 : Gain
  Gain2 : Gain
  "Integrator, Second-Order" : SecondOrderIntegrator  ICSourceX=external  ICSourceDXDT=external
  Interpreted MATLAB Function : MATLABFcn  MATLABFcn=inv  OutputSignalType=real  Output1D=off
  Product : Product  Multiplication=Matrix(*)
  Product1 : Product  Multiplication=Matrix(*)
  Saturation : Saturate  UpperLimit=30  LowerLimit=-30
  Saturation1 : Saturate  UpperLimit=1  LowerLimit=-1
  Sum : Sum  Inputs=|++
  q+delta_q : Outport
  dq+delta_dq : Outport  Port=2
  ddq+delta_ddq : Outport  Port=3
  tau_f_2 : Outport  Port=4
  wires:
  C(q,dq)/1 -> Product/1
  dq/1 -> Product/2
  Product/1 -> Add/1
  g(q)/1 -> Add/2
  Add/1 -> Gain/1
  M(q)/1 -> Interpreted MATLAB Function/1
  Interpreted MATLAB Function/1 -> Product1/1
  Gain/1 -> Add1/1
  tau/1 -> Saturation/1
  Add1/1 -> Product1/2
  Product1/1 -> ddq+delta_ddq/1, "Integrator, Second-Order"/1
  "Integrator, Second-Order"/2 -> Friction/1(dq), dq+delta_dq/1
  "Integrator, Second-Order"/1 -> q+delta_q/1
  q0/1 -> "Integrator, Second-Order"/2
  dq0/1 -> "Integrator, Second-Order"/3
  Sum/1 -> Add1/2
  Saturation/1 -> Sum/1
  Friction/1(tau_f) -> Gain1/1, tau_f_2/1
  Band-Limited White Noise/1 -> Gain2/1
  Saturation1/1 -> Friction/2(d(t))
  Gain1/1 -> Sum/2
  Gain2/1 -> Saturation1/1

== system Dynamics/Subsystem/F gen. ==
  M : Inport
  H : Inport  Port=2
  G : Inport  Port=3
  Z : Inport  Port=4
  Add : Sum  Inputs=+++
  Derivative : Derivative
  Product1 : Product  Multiplication=Matrix(*)
  Product2 : Product  Multiplication=Matrix(*)
  F : Outport
  wires:
  Z/1 -> Product1/2, Derivative/1
  Add/1 -> F/1
  G/1 -> Add/3
  Product2/1 -> Add/1
  M/1 -> Product2/1
  Derivative/1 -> Product2/2
  Product1/1 -> Add/2
  H/1 -> Product1/1

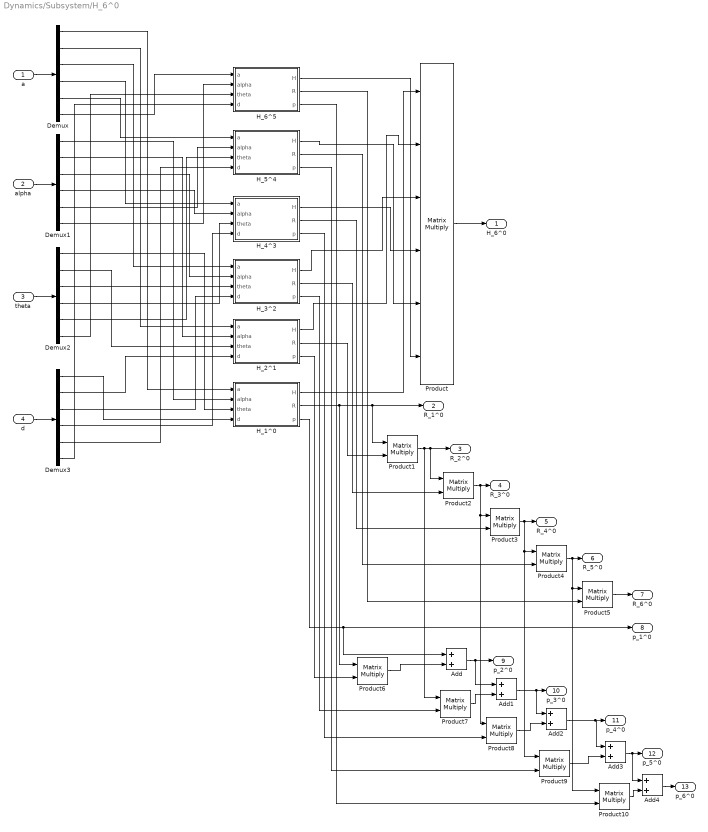
== system Dynamics/Subsystem/H_6^0 ==
  a : Inport
  alpha : Inport  Port=2
  theta : Inport  Port=3
  d : Inport  Port=4
  Add{,1..4} (5 alike) : Sum
  Demux{,1..3} (4 alike) : Demux  Outputs=6
  H_1^0 : Subsystem
  H_2^1 : Subsystem
  H_3^2 : Subsystem
  H_4^3 : Subsystem
  H_5^4 : Subsystem
  H_6^5 : Subsystem
  Product : Product  Inputs=6  Multiplication=Matrix(*)
  Product{1..10} (10 alike) : Product  Multiplication=Matrix(*)
  H_6^0 : Outport
  R_1^0 : Outport  Port=2
  R_2^0 : Outport  Port=3
  R_3^0 : Outport  Port=4
  R_4^0 : Outport  Port=5
  R_5^0 : Outport  Port=6
  R_6^0 : Outport  Port=7
  p_1^0 : Outport  Port=8
  p_2^0 : Outport  Port=9
  p_3^0 : Outport  Port=10
  p_4^0 : Outport  Port=11
  p_5^0 : Outport  Port=12
  p_6^0 : Outport  Port=13
  wires:
  H_6^5/1(H) -> Product/6
  H_5^4/1(H) -> Product/5
  H_2^1/1(H) -> Product/2
  H_1^0/1(H) -> Product/1
  Product/1 -> H_6^0/1
  a/1 -> Demux/1
  d/1 -> Demux3/1
  H_4^3/1(H) -> Product/4
  H_3^2/1(H) -> Product/3
  Product1/1 -> Product7/1, Product2/1, R_2^0/1
  H_2^1/2(R) -> Product1/2
  Product2/1 -> Product8/1, Product3/1, R_3^0/1
  Product3/1 -> Product9/1, Product4/1, R_4^0/1
  Product4/1 -> Product10/1, Product5/1, R_5^0/1
  Product5/1 -> R_6^0/1
  Add/1 -> Add1/1, p_2^0/1
  theta/1 -> Demux2/1
  alpha/1 -> Demux1/1
  Demux/1 -> H_1^0/1(a)
  Demux/6 -> H_6^5/1(a)
  Demux/5 -> H_5^4/1(a)
  Demux/4 -> H_4^3/1(a)
  Demux/3 -> H_3^2/1(a)
  Demux/2 -> H_2^1/1(a)
  Demux1/6 -> H_6^5/2(alpha)
  Demux1/5 -> H_5^4/2(alpha)
  Demux1/4 -> H_4^3/2(alpha)
  Demux1/3 -> H_3^2/2(alpha)
  Demux1/2 -> H_2^1/2(alpha)
  Demux1/1 -> H_1^0/2(alpha)
  Demux2/6 -> H_6^5/3(theta)
  Demux2/5 -> H_5^4/3(theta)
  Demux2/4 -> H_4^3/3(theta)
  Demux2/3 -> H_3^2/3(theta)
  Demux2/2 -> H_2^1/3(theta)
  Demux2/1 -> H_1^0/3(theta)
  Demux3/1 -> H_1^0/4(d)
  Demux3/2 -> H_2^1/4(d)
  Demux3/3 -> H_3^2/4(d)
  Demux3/4 -> H_4^3/4(d)
  Demux3/5 -> H_5^4/4(d)
  Demux3/6 -> H_6^5/4(d)
  H_3^2/2(R) -> Product2/2
  H_4^3/2(R) -> Product3/2
  H_5^4/2(R) -> Product4/2
  H_6^5/2(R) -> Product5/2
  H_1^0/3(p) -> Add/1, p_1^0/1
  H_2^1/3(p) -> Product6/2
  Add1/1 -> Add2/1, p_3^0/1
  H_3^2/3(p) -> Product7/2
  H_4^3/3(p) -> Product8/2
  Add2/1 -> Add3/1, p_4^0/1
  H_5^4/3(p) -> Product9/2
  Add3/1 -> Add4/1, p_5^0/1
  H_6^5/3(p) -> Product10/2
  Add4/1 -> p_6^0/1
  H_1^0/2(R) -> R_1^0/1, Product1/1, Product6/1
  Product6/1 -> Add/2
  Product7/1 -> Add1/2
  Product8/1 -> Add2/2
  Product9/1 -> Add3/2
  Product10/1 -> Add4/2

== system Dynamics/Subsystem/Jacobian ==
  R_1^0 : Inport
  R_2^0 : Inport  Port=2
  R_3^0 : Inport  Port=3
  R_4^0 : Inport  Port=4
  R_5^0 : Inport  Port=5
  R_6^0 : Inport  Port=6
  p_1^0 : Inport  Port=7
  p_2^0 : Inport  Port=8
  p_3^0 : Inport  Port=9
  p_4^0 : Inport  Port=10
  p_5^0 : Inport  Port=11
  p_6^0 : Inport  Port=12
  type1 : Inport  Port=13
  type2 : Inport  Port=14
  type3 : Inport  Port=15
  type4 : Inport  Port=16
  type5 : Inport  Port=17
  type6 : Inport  Port=18
  J(q) gen. : Subsystem
  J_v : Subsystem
  J_w : Subsystem
  Vector Concatenate : Concatenate  Mode=Multidimensional array
  J : Outport
  J(q) : Outport  Port=2
  wires:
  R_1^0/1 -> J_v/1(R_1^0), J_w/1(R_1^0), J(q) gen./1(R_1^0)
  p_1^0/1 -> J_v/7(p_1^0), J(q) gen./7(p_1^0)
  p_2^0/1 -> J_v/8(p_2^0), J(q) gen./8(p_2^0)
  p_3^0/1 -> J_v/9(p_3^0), J(q) gen./9(p_3^0)
  p_4^0/1 -> J_v/10(p_4^0), J(q) gen./10(p_4^0)
  p_5^0/1 -> J_v/11(p_5^0), J(q) gen./11(p_5^0)
  R_2^0/1 -> J_v/2(R_2^0), J_w/2(R_2^0), J(q) gen./2(R_2^0)
  R_3^0/1 -> J_v/3(R_3^0), J_w/3(R_3^0), J(q) gen./3(R_3^0)
  R_4^0/1 -> J_v/4(R_4^0), J_w/4(R_4^0), J(q) gen./4(R_4^0)
  R_5^0/1 -> J_v/5(R_5^0), J_w/5(R_5^0), J(q) gen./5(R_5^0)
  type1/1 -> J_w/7(type1), J_v/13(type1), J(q) gen./12(type1)
  type2/1 -> J_w/8(type2), J(q) gen./13(type2), J_v/14(type2)
  type3/1 -> J_w/9(type3), J(q) gen./14(type3), J_v/15(type3)
  type4/1 -> J_w/10(type4), J(q) gen./15(type4), J_v/16(type4)
  type5/1 -> J_w/11(type5), J_v/17(type5)
  type6/1 -> J_w/12(type6), J_v/18(type6)
  p_6^0/1 -> J_v/12(p_6^0)
  J_v/1(J_v) -> J(q) gen./16(J_v_6(q)), Vector Concatenate/1
  J_w/1(EF J_w) -> Vector Concatenate/2
  Vector Concatenate/1 -> J/1
  J(q) gen./1(J(q)) -> J(q)/1
  J_w/2(J_w1) -> J(q) gen./17(J_w1)
  J_w/3(J_w2) -> J(q) gen./18(J_w2)
  J_w/4(J_w3) -> J(q) gen./19(J_w3)
  J_w/5(J_w4) -> J(q) gen./20(J_w4)
  J_w/6(J_w5) -> J(q) gen./21(J_w5)
  J_w/7(J_w6) -> J(q) gen./22(J_w6)
  R_6^0/1 -> J_v/6(R_6^0), J_w/6(R_6^0), J(q) gen./6(R_6^0)

== system Dynamics/Subsystem/M(q),C(q,dq),g(q) ==
  m : Inport
  J(q) : Inport  Port=2
  I1 : Inport  Port=3
  I2 : Inport  Port=4
  I3 : Inport  Port=5
  I4 : Inport  Port=6
  I5 : Inport  Port=7
  I6 : Inport  Port=8
  w1 : Inport  Port=9
  w2 : Inport  Port=10
  w3 : Inport  Port=11
  w4 : Inport  Port=12
  w5 : Inport  Port=13
  w6 : Inport  Port=14
  Add : Sum
  G gen : Subsystem
  Interpreted MATLAB Function : MATLABFcn  MATLABFcn=transpose  OutputSignalType=real  Output1D=off
  M,H : Subsystem
  Product{,1..3} (4 alike) : Product  Multiplication=Matrix(*)
  Product4 : Product  Inputs=3  Multiplication=Matrix(*)
  dJ : Derivative
  g(q) : Outport
  C(q,dq) : Outport  Port=2
  M(q) : Outport  Port=3
  M : Outport  Port=4
  H : Outport  Port=5
  G : Outport  Port=6
  wires:
  J(q)/1 -> Interpreted MATLAB Function/1, Product4/3, Product2/2, dJ/1
  Interpreted MATLAB Function/1 -> Product4/1, Product3/1, Product/1
  Product/1 -> g(q)/1
  m/1 -> G gen/1(m), M,H/1(m)
  I1/1 -> M,H/2(I1)
  I2/1 -> M,H/3(I2)
  I3/1 -> M,H/4(I3)
  I4/1 -> M,H/5(I4)
  I5/1 -> M,H/6(I5)
  I6/1 -> M,H/7(I6)
  w1/1 -> M,H/8(w1)
  w2/1 -> M,H/9(w2)
  w3/1 -> M,H/10(w3)
  w4/1 -> M,H/11(w4)
  w5/1 -> M,H/12(w5)
  w6/1 -> M,H/13(w6)
  M,H/1(M) -> Product1/1, M/1, Product4/2
  dJ/1 -> Product1/2
  M,H/2(H) -> H/1, Product2/1
  Product1/1 -> Add/1
  Product2/1 -> Add/2
  Add/1 -> Product3/2
  Product3/1 -> C(q,dq)/1
  Product4/1 -> M(q)/1
  G gen/1(G) -> G/1, Product/2

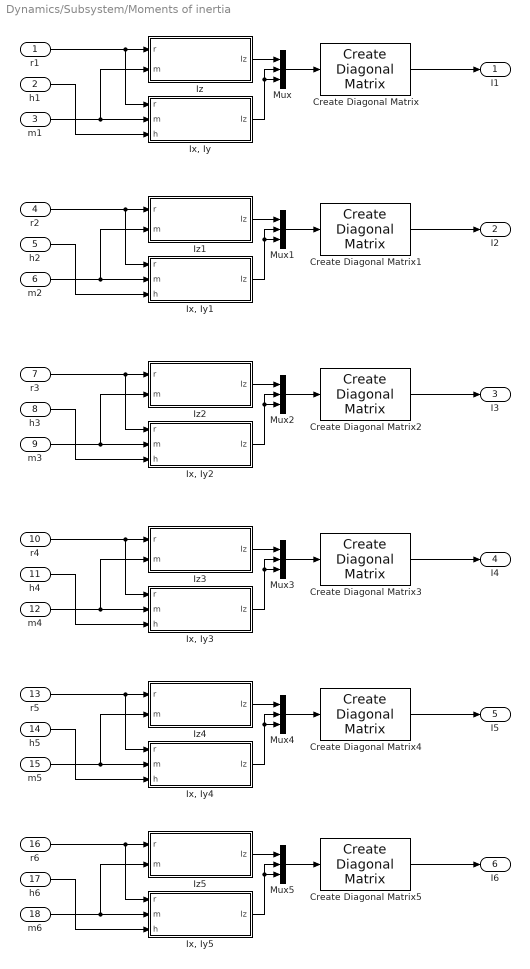
== system Dynamics/Subsystem/Moments of inertia ==
  r1 : Inport
  h1 : Inport  Port=2
  m1 : Inport  Port=3
  r2 : Inport  Port=4
  h2 : Inport  Port=5
  m2 : Inport  Port=6
  r3 : Inport  Port=7
  h3 : Inport  Port=8
  m3 : Inport  Port=9
  r4 : Inport  Port=10
  h4 : Inport  Port=11
  m4 : Inport  Port=12
  r5 : Inport  Port=13
  h5 : Inport  Port=14
  m5 : Inport  Port=15
  r6 : Inport  Port=16
  h6 : Inport  Port=17
  m6 : Inport  Port=18
  Create Diagonal Matrix{,1..5} (6 alike) : dspmtrx3/Create Diagonal Matrix
  "Ix, Iy" : Subsystem
  "Ix, Iy1" : Subsystem
  "Ix, Iy2" : Subsystem
  "Ix, Iy3" : Subsystem
  "Ix, Iy4" : Subsystem
  "Ix, Iy5" : Subsystem
  Iz : Subsystem
  Iz1 : Subsystem
  Iz2 : Subsystem
  Iz3 : Subsystem
  Iz4 : Subsystem
  Iz5 : Subsystem
  Mux{,1..5} (6 alike) : Mux  Inputs=3
  I1 : Outport
  I2 : Outport  Port=2
  I3 : Outport  Port=3
  I4 : Outport  Port=4
  I5 : Outport  Port=5
  I6 : Outport  Port=6
  wires:
  r1/1 -> "Ix, Iy"/1(r), Iz/1(r)
  m1/1 -> "Ix, Iy"/2(m), Iz/2(m)
  h1/1 -> "Ix, Iy"/3(h)
  Mux/1 -> Create Diagonal Matrix/1
  Iz/1(Iz) -> Mux/1
  "Ix, Iy"/1(Iz) -> Mux/3, Mux/2
  Create Diagonal Matrix/1 -> I1/1
  r2/1 -> "Ix, Iy1"/1(r), Iz1/1(r)
  m2/1 -> "Ix, Iy1"/2(m), Iz1/2(m)
  h2/1 -> "Ix, Iy1"/3(h)
  Mux1/1 -> Create Diagonal Matrix1/1
  Iz1/1(Iz) -> Mux1/1
  "Ix, Iy1"/1(Iz) -> Mux1/3, Mux1/2
  Create Diagonal Matrix1/1 -> I2/1
  r3/1 -> "Ix, Iy2"/1(r), Iz2/1(r)
  m3/1 -> "Ix, Iy2"/2(m), Iz2/2(m)
  h3/1 -> "Ix, Iy2"/3(h)
  Mux2/1 -> Create Diagonal Matrix2/1
  Iz2/1(Iz) -> Mux2/1
  "Ix, Iy2"/1(Iz) -> Mux2/3, Mux2/2
  Create Diagonal Matrix2/1 -> I3/1
  r4/1 -> "Ix, Iy3"/1(r), Iz3/1(r)
  m4/1 -> "Ix, Iy3"/2(m), Iz3/2(m)
  h4/1 -> "Ix, Iy3"/3(h)
  Mux3/1 -> Create Diagonal Matrix3/1
  Iz3/1(Iz) -> Mux3/1
  "Ix, Iy3"/1(Iz) -> Mux3/3, Mux3/2
  Create Diagonal Matrix3/1 -> I4/1
  r5/1 -> "Ix, Iy4"/1(r), Iz4/1(r)
  m5/1 -> "Ix, Iy4"/2(m), Iz4/2(m)
  h5/1 -> "Ix, Iy4"/3(h)
  Mux4/1 -> Create Diagonal Matrix4/1
  Iz4/1(Iz) -> Mux4/1
  "Ix, Iy4"/1(Iz) -> Mux4/3, Mux4/2
  Create Diagonal Matrix4/1 -> I5/1
  r6/1 -> "Ix, Iy5"/1(r), Iz5/1(r)
  m6/1 -> "Ix, Iy5"/2(m), Iz5/2(m)
  h6/1 -> "Ix, Iy5"/3(h)
  Mux5/1 -> Create Diagonal Matrix5/1
  Iz5/1(Iz) -> Mux5/1
  "Ix, Iy5"/1(Iz) -> Mux5/3, Mux5/2
  Create Diagonal Matrix5/1 -> I6/1

== system Dynamics/Subsystem/Slotine ==
  g(q) : Inport
  C(q,dq) : Inport  Port=2
  M(q) : Inport  Port=3
  q_d : Inport  Port=4
  dq_d : Inport  Port=5
  ddq_d : Inport  Port=6
  q : Inport  Port=7
  dq : Inport  Port=8
  Lambda : Inport  Port=9
  K : Inport  Port=10
  Clock : Clock
  Gain : Gain  Gain=-1
  Math Function : Math  SignedPower=on
  S-gen : Subsystem
  V-gen : Subsystem
  dV-gen : Subsystem
  dq_tilde : Sum  Inputs=-+
  q_tilde : Sum  Inputs=-+
  tau-gen : Subsystem
  u0-gen : Subsystem
  tau : Outport
  S : Outport  Port=2
  wires:
  q_d/1 -> q_tilde/1
  q/1 -> q_tilde/2
  dq_d/1 -> V-gen/2(dq_d), dq_tilde/1
  dq/1 -> S-gen/1(dq), dq_tilde/2
  ddq_d/1 -> dV-gen/2(ddq_d)
  q_tilde/1 -> V-gen/1(q_tilde)
  Lambda/1 -> dV-gen/3(Gamma), V-gen/3(Gamma)
  dq_tilde/1 -> dV-gen/1(dq_tilde)
  V-gen/1(V) -> tau-gen/4(V), S-gen/2(V)
  M(q)/1 -> tau-gen/1(M)
  C(q,dq)/1 -> tau-gen/2(C)
  g(q)/1 -> tau-gen/3(g)
  dV-gen/1(dV) -> tau-gen/5(dV)
  S-gen/1(S) -> u0-gen/1(S), S/1, tau-gen/6(S)
  K/1 -> tau-gen/7(K)
  tau-gen/1(tau) -> tau/1
  u0-gen/1(u0) -> tau-gen/8(u0)
  Math Function/1 -> u0-gen/2(sigma(t))
  Clock/1 -> Gain/1
  Gain/1 -> Math Function/1
